simulink model "parallel_two_levelsvpwm"  (R2016a)
settings: Solver=VariableStepAuto  StartTime=0.0  StopTime=0.5  RelTol=1e-3
libraries: powerlib x50, simulink x7, powerlib_meascontrol x2
settings Model: Creator=hakan  LastModifiedBy=hakan
settings DataIOCC: LimitDataPoints=on
settings DebuggingCC: AllowSymbolicDim=off
settings ModelReferenceCC: PropagateSignalLabelsOutOfModel=off
settings GRTTargetCC: GeneratePreprocessorConditionals=Use local settings

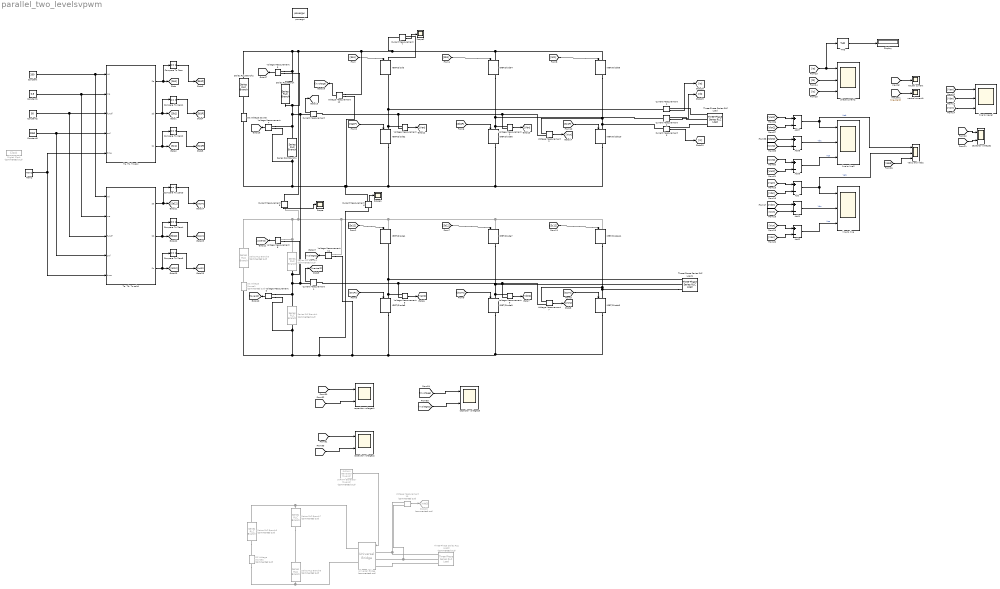
== system parallel_two_levelsvpwm ==
  Add{,1..2,7..9} (6 alike) : Sum  Inputs=+-
  Compare To Zero{,1..5} (6 alike) : simulink/Logic and Bit Operations/Compare To Zero  relop===  OutDataTypeStr=boolean
  Constant : Constant  Value=200
  Constant1 : Constant  Value=0.8
  Constant2 : Constant  Value=50
  Constant3 : Constant  Value=2050  VectorParams1D=off
  Current Measurement{,1..7} (8 alike) : powerlib/Measurements/Current Measurement  PhasorSimulation=off  OutputType=Complex  PSBequivalent=0
  DC Voltage Source : powerlib/Electrical Sources/DC Voltage Source  Amplitude=540  Measurements=None
  DC Voltage Source1 : powerlib/Electrical Sources/DC Voltage Source  Commented=on  Amplitude=540  Measurements=None
  DC Voltage Source2 : powerlib/Electrical Sources/DC Voltage Source  Commented=on  Amplitude=540  Measurements=None
  Digital Clock : DigitalClock  Commented=on  SampleTime=0.0000001
  Display : Display
  Goto28 : Goto  Commented=on  GotoTag=Vab3
  IGBT/Diode{,1..11} (12 alike) : powerlib/Power Electronics/IGBT//Diode  Ron=1e-3  Rs=1e5  Cs=inf  Measurements=on
  Ramp : simulink/Sources/Ramp  slope=1  start=0  X0=0
  SVPWM Generator (2-Level) : powerlib_meascontrol/Pulse & Signal Generators/SVPWM Generator (2-Level)  Commented=on  InputType=Internally generated  SwitchingPattern=Pattern #1  Fc=2050  ParUref="[0.8 0  50]"  Ts=0
  Scope : Scope
  Scope1 : Scope
  Scope2 : Scope
  Series RLC Branch : powerlib/Elements/Series RLC Branch  LConnTagsString=__new0  RConnTagsString=__new0  BranchType=C  Resistance=1  Inductance=1e-3  SetiL0=off  InitialCurrent=0  Capacitance=10e-6  Setx0=off  InitialVoltage=0  Measurements=None
  Series RLC Branch1 : powerlib/Elements/Series RLC Branch  LConnTagsString=__new0  RConnTagsString=__new0  BranchType=C  Resistance=1  Inductance=1e-3  SetiL0=off  InitialCurrent=0  Capacitance=10e-6  Setx0=off  InitialVoltage=0  Measurements=None
  Series RLC Branch2 : powerlib/Elements/Series RLC Branch  LConnTagsString=__new0  RConnTagsString=__new0  BranchType=R  Resistance=1  Inductance=1e-3  SetiL0=off  InitialCurrent=0  Capacitance=1000e-6  Setx0=off  InitialVoltage=0  Measurements=None
  Series RLC Branch3 : powerlib/Elements/Series RLC Branch  Commented=on  LConnTagsString=__new0  RConnTagsString=__new0  BranchType=C  Resistance=1  Inductance=1e-3  SetiL0=off  InitialCurrent=0  Capacitance=10e-6  Setx0=off  InitialVoltage=0  Measurements=None
  Series RLC Branch4 : powerlib/Elements/Series RLC Branch  Commented=on  LConnTagsString=__new0  RConnTagsString=__new0  BranchType=C  Resistance=1  Inductance=1e-3  SetiL0=off  InitialCurrent=0  Capacitance=10e-6  Setx0=off  InitialVoltage=0  Measurements=None
  Series RLC Branch5 : powerlib/Elements/Series RLC Branch  Commented=on  LConnTagsString=__new0  RConnTagsString=__new0  BranchType=R  Resistance=1  Inductance=1e-3  SetiL0=off  InitialCurrent=0  Capacitance=1000e-6  Setx0=off  InitialVoltage=0  Measurements=None
  Series RLC Branch6 : powerlib/Elements/Series RLC Branch  Commented=on  LConnTagsString=__new0  RConnTagsString=__new0  BranchType=R  Resistance=1  Inductance=1e-3  SetiL0=off  InitialCurrent=0  Capacitance=1000e-6  Setx0=off  InitialVoltage=0  Measurements=None
  Series RLC Branch7 : powerlib/Elements/Series RLC Branch  Commented=on  LConnTagsString=__new0  RConnTagsString=__new0  BranchType=C  Resistance=1  Inductance=1e-3  SetiL0=off  InitialCurrent=0  Capacitance=20e-6  Setx0=off  InitialVoltage=0  Measurements=None
  Series RLC Branch8 : powerlib/Elements/Series RLC Branch  Commented=on  LConnTagsString=__new0  RConnTagsString=__new0  BranchType=C  Resistance=1  Inductance=1e-3  SetiL0=off  InitialCurrent=0  Capacitance=20e-6  Setx0=off  InitialVoltage=0  Measurements=None
  THD : powerlib_meascontrol/Measurements/THD  Freq=50  Ts=0
  "Ta, Tb, Tc calc" : MATLAB Function  TreatAsAtomicUnit=on
  "Ta, Tb, Tc calc1" : MATLAB Function  TreatAsAtomicUnit=on
  Three-Phase Series RLC Load : powerlib/Elements/Three-Phase Series RLC Load  LConnTagsString=A|B|C  Configuration=Y (floating)  NominalVoltage=1000  Vabc=[1e3 1e3 1e3]  Vabcp=[1e3 1e3 1e3]  NominalFrequency=50  UnbalancedPower=off  ActivePower=8000/2  InductivePower=3870/2  CapacitivePower=0  Pabc=[10e3 9e3 11e3]  QLabc=[100 90 110]  QCabc=[100 90 110]  Pabcp=[10e3 9e3 11e3]  QLabcp=[100 90 110]  QCabcp=[100 90 110]  Measurements=None  LoadType=constant Z
  Three-Phase Series RLC Load1 : powerlib/Elements/Three-Phase Series RLC Load  LConnTagsString=A|B|C  Configuration=Y (floating)  NominalVoltage=1000  Vabc=[1e3 1e3 1e3]  Vabcp=[1e3 1e3 1e3]  NominalFrequency=50  UnbalancedPower=off  ActivePower=8000/2  InductivePower=3870/2  CapacitivePower=0  Pabc=[10e3 9e3 11e3]  QLabc=[100 90 110]  QCabc=[100 90 110]  Pabcp=[10e3 9e3 11e3]  QLabcp=[100 90 110]  QCabcp=[100 90 110]  Measurements=None  LoadType=constant Z
  Three-Phase Series RLC Load2 : powerlib/Elements/Three-Phase Series RLC Load  Commented=on  LConnTagsString=A|B|C  Configuration=Y (floating)  NominalVoltage=1000  Vabc=[1e3 1e3 1e3]  Vabcp=[1e3 1e3 1e3]  NominalFrequency=50  UnbalancedPower=off  ActivePower=8000/2  InductivePower=3870/2  CapacitivePower=0  Pabc=[10e3 9e3 11e3]  QLabc=[100 90 110]  QCabc=[100 90 110]  Pabcp=[10e3 9e3 11e3]  QLabcp=[100 90 110]  QCabcp=[100 90 110]  Measurements=None  LoadType=constant Z
  Universal Bridge : powerlib/Power Electronics/Universal Bridge  Commented=on  Arms=3  SnubberResistance=1e5  SnubberCapacitance=inf  Device=IGBT / Diodes  Ron=1e-3  Lon=0  ForwardVoltages="[  0  0  ]"  ForwardVoltage=0  GTOparameters=[ 10e-6 , 20e-6 ]  IGBTparameters=[ 1e-6 , 2e-6 ]  Measurements=None  Measurements_2=None  converterType=Rectifier
  Vab1 and Vab2 : Scope  NumInputPorts=3
  Voltage Measurement{,1..9,11..12} (12 alike) : powerlib/Measurements/Voltage Measurement  PhasorSimulation=off  OutputType=Complex  PSBequivalent=0
  Voltage Measurement10 : powerlib/Measurements/Voltage Measurement  Commented=on  PhasorSimulation=off  OutputType=Complex  PSBequivalent=0
  capacitor voltages{,1..3} (4 alike) : Scope  NumInputPorts=2
  line to line : Scope  NumInputPorts=3
  line to line2 : Scope  NumInputPorts=3
  line to neural : Scope  NumInputPorts=3
  neutral current : Scope
  neutral current1 : Scope
  phase currents : Scope  NumInputPorts=3
  powergui : powerlib/powergui  Priority=1  SimulationMode=Discrete  SolverType=Tustin/Backward Euler (TBE)  SampleTime=50e-8  frequency=60  SPID=off  DisableSnubberDevices=off  DisableRonSwitches=off  DisableVfSwitches=off  SwTol=0  DisplayEquations=off  Interpol=off  ExternalGateDelay=off  methode=off  Ts=10  FunctionMessages=off  echomessages=off  HookPort=off  EnableUseOfTLC=off  x0status=blocks  frequencyindice=0  Pbase=100e6  ErrMax=1e-4  Iterations=50  UnitsV=kV  UnitsW=MW  buscounter=0  RestoreLinks=warning  ResistiveCurrentMeasurement=off  Frange=[0:2:500]  Ylog=off  Xlog=on  ShowGrid=off  save=off  variable=ZData  structure=linetoline  ZoomFFT=off  StartTime=0.0  cycles=2  DisplayStyle=1  fundamental=50  FreqAxis=off  MaxFrequency=5000  frequencyindicesteady=1  RmsSteady=1  display=off
  wires:
  "Ta, Tb, Tc calc"/1(Sa) -> Compare To Zero/1, [Sa1]
  "Ta, Tb, Tc calc"/2(Sb) -> Compare To Zero1/1, [Sb1]
  "Ta, Tb, Tc calc"/3(Sc) -> Compare To Zero2/1, [Sc1]
  Compare To Zero/1 -> [Sa1P]
  Compare To Zero1/1 -> [Sb1P]
  Compare To Zero2/1 -> [Sc1P]
  Constant/1 -> "Ta, Tb, Tc calc1"/1(Vd), "Ta, Tb, Tc calc"/1(Vd)
  Constant1/1 -> "Ta, Tb, Tc calc1"/2(ma), "Ta, Tb, Tc calc"/2(ma)
  Constant2/1 -> "Ta, Tb, Tc calc1"/3(fundf), "Ta, Tb, Tc calc"/3(fundf)
  Constant3/1 -> "Ta, Tb, Tc calc1"/4(swf), "Ta, Tb, Tc calc"/4(swf)
  Ramp/1 -> "Ta, Tb, Tc calc"/5(time), "Ta, Tb, Tc calc1"/5(time)
  [Ineutral] -> neutral current/1
  [Ib] -> phase currents/2
  [Ic] -> phase currents/3
  [Van] -> Add/1
  [Vbn] -> Add/2
  Add/1 -> Vab1 and Vab2/2, line to line/1  "Vab"
  [Vbn] -> Add1/1
  [Vcn] -> Add1/2
  Add1/1 -> line to line/2  "Vbc"
  [Vcn] -> Add2/1
  [Van] -> Add2/2
  Add2/1 -> line to line/3  "Vca"
  [Van] -> line to neural/1
  [Vbn] -> line to neural/2
  [Vcn] -> line to neural/3
  [lowerc] -> capacitor voltages/2
  [upperc] -> capacitor voltages/1
  [Sa1] -> IGBT/Diode/1
  [Sa1P] -> IGBT/Diode2/1
  [Sb1] -> IGBT/Diode4/1
  [Sb1P] -> IGBT/Diode6/1
  [Sc1] -> IGBT/Diode8/1
  [Sc1P] -> IGBT/Diode10/1
  Voltage Measurement/1 -> [Van]
  Voltage Measurement1/1 -> [Vbn]
  Voltage Measurement2/1 -> [Vcn]
  Voltage Measurement3/1 -> [upperc]
  Voltage Measurement4/1 -> [lowerc]
  Current Measurement/1 -> [Ineutral]
  Current Measurement1/1 -> [Ia]
  Current Measurement2/1 -> [Ib]
  Current Measurement3/1 -> [Ic]
  "Ta, Tb, Tc calc1"/1(Sa) -> [Sa12], Compare To Zero3/1
  "Ta, Tb, Tc calc1"/2(Sb) -> [Sb12], Compare To Zero4/1
  "Ta, Tb, Tc calc1"/3(Sc) -> [Sc12], Compare To Zero5/1
  Compare To Zero3/1 -> [Sa1P2]
  Compare To Zero4/1 -> [Sb1P2]
  Compare To Zero5/1 -> [Sc1P2]
  [Sa12] -> IGBT/Diode1/1
  [Sa1P2] -> IGBT/Diode5/1
  [Sb12] -> IGBT/Diode7/1
  [Sb1P2] -> IGBT/Diode9/1
  [Sc12] -> IGBT/Diode11/1
  [Sc1P2] -> IGBT/Diode3/1
  Voltage Measurement5/1 -> [Van2]
  Voltage Measurement6/1 -> [Vbn2]
  Voltage Measurement7/1 -> [Vcn2]
  Voltage Measurement8/1 -> [upperc2]
  Voltage Measurement9/1 -> [lowerc2]
  Current Measurement4/1 -> [Ineutral2]
  Voltage Measurement11/1 -> [involtage2]
  [Van2] -> Add7/1
  [Vbn2] -> Add7/2
  Add7/1 -> Vab1 and Vab2/1, line to line2/1  "Vab"
  [Vbn2] -> Add8/1
  [Vcn2] -> Add8/2
  Add8/1 -> line to line2/2  "Vbc"
  [Vcn2] -> Add9/1
  [Van2] -> Add9/2
  Add9/1 -> line to line2/3  "Vca"
  [upperc] -> capacitor voltages1/1
  [lowerc] -> capacitor voltages2/1
  [upperc2] -> capacitor voltages1/2
  [lowerc2] -> capacitor voltages2/2
  [involtage] -> capacitor voltages3/1
  [involtage2] -> capacitor voltages3/2
  [Ineutral2] -> neutral current1/1
  SVPWM Generator (2-Level)/1 -> Universal Bridge/1
  Voltage Measurement10/1 -> Goto28/1
  [Vab3] -> Vab1 and Vab2/3
  Voltage Measurement12/1 -> [involtage]
  [Ia] -> THD/1, phase currents/1
  THD/1 -> Display/1
  Current Measurement5/1 -> Scope/1
  Current Measurement6/1 -> Scope1/1
  Current Measurement7/1 -> Scope2/1
  connections:
  Series RLC Branch5/LConn1 -- Voltage Measurement11/LConn1 -- IGBT/Diode1/LConn1 -- IGBT/Diode11/LConn1 -- IGBT/Diode7/LConn1 -- Current Measurement5/RConn1 -- Voltage Measurement8/LConn1 -- Series RLC Branch3/LConn1
  Current Measurement1/LConn1 -- IGBT/Diode/RConn1 -- IGBT/Diode2/LConn1 -- Voltage Measurement/LConn1
  Current Measurement/LConn1 -- Voltage Measurement/LConn2 -- Voltage Measurement2/LConn2 -- Voltage Measurement1/LConn2
  Current Measurement2/LConn1 -- IGBT/Diode4/RConn1 -- IGBT/Diode6/LConn1 -- Voltage Measurement1/LConn1
  Voltage Measurement2/LConn1 -- IGBT/Diode10/LConn1 -- Current Measurement3/LConn1 -- IGBT/Diode8/RConn1
  Three-Phase Series RLC Load/LConn3 -- Current Measurement3/RConn1
  Three-Phase Series RLC Load/LConn1 -- Current Measurement1/RConn1
  Three-Phase Series RLC Load/LConn2 -- Current Measurement2/RConn1
  DC Voltage Source/RConn1 -- Series RLC Branch2/RConn1
  IGBT/Diode5/LConn1 -- IGBT/Diode1/RConn1 -- Three-Phase Series RLC Load1/LConn1 -- Voltage Measurement5/LConn1
  Voltage Measurement7/LConn2 -- Voltage Measurement6/LConn2 -- Current Measurement4/LConn1 -- Voltage Measurement5/LConn2
  IGBT/Diode9/LConn1 -- IGBT/Diode7/RConn1 -- Three-Phase Series RLC Load1/LConn2 -- Voltage Measurement6/LConn1
  Three-Phase Series RLC Load1/LConn3 -- IGBT/Diode3/LConn1 -- Voltage Measurement7/LConn1 -- IGBT/Diode11/RConn1
  DC Voltage Source1/RConn1 -- Series RLC Branch5/RConn1
  Current Measurement6/RConn1 -- IGBT/Diode2/RConn1 -- IGBT/Diode10/RConn1 -- IGBT/Diode6/RConn1 -- Voltage Measurement12/LConn2 -- Series RLC Branch1/RConn1 -- Voltage Measurement4/LConn2 -- DC Voltage Source/LConn1
  Three-Phase Series RLC Load2/LConn1 -- Universal Bridge/LConn1 -- Voltage Measurement10/LConn1
  Three-Phase Series RLC Load2/LConn2 -- Universal Bridge/LConn2 -- Voltage Measurement10/LConn2
  Three-Phase Series RLC Load2/LConn3 -- Universal Bridge/LConn3
  Series RLC Branch6/RConn1 -- DC Voltage Source2/RConn1
  Series RLC Branch7/RConn1 -- Series RLC Branch8/LConn1
  Series RLC Branch6/LConn1 -- Universal Bridge/RConn1 -- Series RLC Branch7/LConn1
  DC Voltage Source2/LConn1 -- Universal Bridge/RConn2 -- Series RLC Branch8/RConn1
  Voltage Measurement8/LConn2 -- Series RLC Branch3/RConn1 -- Current Measurement4/RConn1 -- Series RLC Branch/RConn1 -- Voltage Measurement3/LConn2 -- Voltage Measurement4/LConn1 -- Series RLC Branch1/LConn1 -- Current Measurement/RConn1 -- Voltage Measurement9/LConn1 -- Series RLC Branch4/LConn1
  Voltage Measurement11/LConn2 -- Voltage Measurement9/LConn2 -- Series RLC Branch4/RConn1 -- DC Voltage Source1/LConn1 -- Current Measurement6/LConn1 -- IGBT/Diode9/RConn1 -- IGBT/Diode3/RConn1 -- IGBT/Diode5/RConn1
  IGBT/Diode/LConn1 -- Current Measurement7/RConn1
  Voltage Measurement12/LConn1 -- Current Measurement7/LConn1 -- IGBT/Diode4/LConn1 -- IGBT/Diode8/LConn1 -- Current Measurement5/LConn1 -- Series RLC Branch2/LConn1 -- Voltage Measurement3/LConn1 -- Series RLC Branch/LConn1

== matlab function parallel_two_levelsvpwm/Ta, Tb, Tc calc ==
  data: Sa output; Sb output; Vd input; ma input; fundf input; swf input; time input; Sc output
function [Sa, Sb, Sc] = fcn(Vd,ma,fundf, swf, time)
% this program works for magnitude of Vref is greater then Vd/3 meaning ma
% must be greater than 1/sqrt(3). for smaller ma's computation is a bit
% more tricky therefore it is omitted for simplicity for now. 
Vref = ma*Vd/sqrt(3); %magnitude of Vref
theta = 2*pi*fundf*time; %angle of Vref
angle = mod(theta, 2*pi);
Ts = 1/swf;
Ta = 0;
Tb = 0;
Tc = 0;
T0 = 0;
n=0;
output = 0;
%Sector1 = 0; Sector2 = 0; Sector3 = 0; Sector4= 0; Sector5 = 0; Sector6 = 0;
Sa=0; Sb=0; Sc=0;
timee = mod(time,Ts);



%% Sector 1
if (angle<=pi/3)&&(angle>0)  % sector 1
    n = 1;
    thetaprime = angle - (n-1)*pi/3;
    
    Ta = Ts*ma*sin(pi/3-thetaprime);
    Tb = Ts*ma*sin(thetaprime);
    T0 = Ts-Ta-Tb;
    
    times = [T0/4 Tb/2 Ta/2 T0/2 Ta/2 Tb/2 T0/4];
    times = cumsum(times);
    va= [0 1 1 1 1 1 0];
    vb= [0 0 1 1 1 0 0];
    vc= [0 0 0 1 0 0 0];
    
    for j = 1:7            
            if(timee<times(j))
                break
            end
    end
        Sa=va(j); 
        Sb=vb(j); 
        Sc=vc(j); 
end
%% Sector 2
if (angle<=2*pi/3)&&(angle>pi/3)  % sector 2
    n = 2;
    thetaprime = angle - (n-1)*pi/3;
    
    Ta = Ts*ma*sin(pi/3-thetaprime);
    Tb = Ts*ma*sin(thetaprime);
    T0 = Ts-Ta-Tb;   
    
    times = [T0/4 Tb/2 Ta/2 T0/2 Ta/2 Tb/2 T0/4];
    times = cumsum(times);
    va= [0 0 1 1 1 0 0];
    vb= [0 1 1 1 1 1 0];
    vc= [0 0 0 1 0 0 0];
    
    for j = 1:7            
            if(timee<times(j))
                break
            end
    end
        Sa=va(j); 
        Sb=vb(j); 
        Sc=vc(j); 
end


%% Sector 3
if (angle<=pi)&&(angle>2*pi/3)  % sector 3
    n = 3;
    thetaprime = angle - (n-1)*pi/3;
    
    Ta = Ts*ma*sin(pi/3-thetaprime);
    Tb = Ts*ma*sin(thetaprime);
    T0 = Ts-Ta-Tb;  
    
    times = [T0/4 Tb/2 Ta/2 T0/2 Ta/2 Tb/2 T0/4];
    times = cumsum(times);
    va= [0 0 0 1 0 0 0];
    vb= [0 1 1 1 1 1 0];
    vc= [0 0 1 1 1 0 0];
    
    for j = 1:7            
            if(timee<times(j))
                break
            end
    end
        Sa=va(j); 
        Sb=vb(j); 
        Sc=vc(j);     
end


%% Sector 4
if (angle<=4*pi/3)&&(angle>pi)  % sector 4
    n = 4;
    thetaprime = angle - (n-1)*pi/3;
    
    Ta = Ts*ma*sin(pi/3-thetaprime);
    Tb = Ts*ma*sin(thetaprime);
    T0 = Ts-Ta-Tb;
    
    times = [T0/4 Tb/2 Ta/2 T0/2 Ta/2 Tb/2 T0/4];
    times = cumsum(times);
    va = [0 0 0 1 0 0 0];
    vb = [0 0 1 1 1 0 0];
    vc = [0 1 1 1 1 1 0];
    
    for j = 1:7            
            if(timee<times(j))
                break
            end
    end
        Sa=va(j); 
        Sb=vb(j); 
        Sc=vc(j); 
    
end


%% Sector 5 
if (angle<=5*pi/3)&&(angle>4*pi/3)  % sector 5
    n = 5;
    thetaprime = angle - (n-1)*pi/3;
    
    Ta = Ts*ma*sin(pi/3-thetaprime);
    Tb = Ts*ma*sin(thetaprime);
    T0 = Ts-Ta-Tb;
    
    times = [T0/4 Tb/2 Ta/2 T0/2 Ta/2 Tb/2 T0/4];
    times = cumsum(times);
    va= [0 0 1 1 1 0 0];
    vb= [0 0 0 1 0 0 0];
    vc= [0 1 1 1 1 1 0];
    
    for j = 1:7            
            if(timee<times(j))
                break
            end
    end
        Sa=va(j); 
        Sb=vb(j); 
        Sc=vc(j); 
    
end


%% Sector 6 
if (angle<=2*pi)&&(angle>5*pi/3)  % sector 6
    n = 6;
    thetaprime = angle - (n-1)*pi/3;
    
    Ta = Ts*ma*sin(pi/3-thetaprime);
    Tb = Ts*ma*sin(thetaprime);
    T0 = Ts-Ta-Tb;
    
    times = [T0/4 Tb/2 Ta/2 T0/2 Ta/2 Tb/2 T0/4];
    times = cumsum(times);
    va= [0 1 1 1 1 1 0];
    vb= [0 0 0 1 0 0 0];
    vc= [0 0 1 1 1 0 0];
    
    
    for j = 1:7            
            if(timee<times(j))
                break
            end
    end
        Sa=va(j); 
        Sb=vb(j); 
        Sc=vc(j); 
end

== matlab function parallel_two_levelsvpwm/Ta, Tb, Tc calc1 ==
  data: Sa output; Sb output; Vd input; ma input; fundf input; swf input; time input; Sc output
function [Sa, Sb, Sc] = fcn(Vd,ma,fundf, swf, time)
% this program works for magnitude of Vref is greater then Vd/3 meaning ma
% must be greater than 1/sqrt(3). for smaller ma's computation is a bit
% more tricky therefore it is omitted for simplicity for now. 
Vref = ma*Vd/sqrt(3); %magnitude of Vref
theta = 2*pi*fundf*time; %angle of Vref
angle = mod(theta, 2*pi);
Ts = 1/swf;
Ta = 0;
Tb = 0;
Tc = 0;
T0 = 0;
n=0;
output = 0;
%Sector1 = 0; Sector2 = 0; Sector3 = 0; Sector4= 0; Sector5 = 0; Sector6 = 0;
Sa=0; Sb=0; Sc=0;
timee = mod(time+Ts/4,Ts);



%% Sector 1
if (mod(theta, 2*pi)<=pi/3)&&(mod(theta, 2*pi)>0)  % sector 1
    n = 1;
    thetaprime = angle - (n-1)*pi/3;
    
    Ta = Ts*ma*sin(pi/3-thetaprime);
    Tb = Ts*ma*sin(thetaprime);
    T0 = Ts-Ta-Tb;
    
    times = [T0/4 Tb/2 Ta/2 T0/2 Ta/2 Tb/2 T0/4];
    times = cumsum(times);
    va= [0 1 1 1 1 1 0];
    vb= [0 0 1 1 1 0 0];
    vc= [0 0 0 1 0 0 0];
    
    for j = 1:7            
            if(timee<times(j))
                break
            end
    end
        Sa=va(j); 
        Sb=vb(j); 
        Sc=vc(j); 
end
%% Sector 2
if (mod(theta, 2*pi)<=2*pi/3)&&(mod(theta, 2*pi)>pi/3)  % sector 2
    n = 2;
    thetaprime = angle - (n-1)*pi/3;
    
    Ta = Ts*ma*sin(pi/3-thetaprime);
    Tb = Ts*ma*sin(thetaprime);
    T0 = Ts-Ta-Tb;   
    
    times = [T0/4 Tb/2 Ta/2 T0/2 Ta/2 Tb/2 T0/4];
    times = cumsum(times);
    va= [0 0 1 1 1 0 0];
    vb= [0 1 1 1 1 1 0];
    vc= [0 0 0 1 0 0 0];
    
    for j = 1:7            
            if(timee<times(j))
                break
            end
    end
        Sa=va(j); 
        Sb=vb(j); 
        Sc=vc(j); 
end


%% Sector 3
if (mod(theta, 2*pi)<=pi)&&(mod(theta, 2*pi)>2*pi/3)  % sector 3
    n = 3;
    thetaprime = angle - (n-1)*pi/3;
    
    Ta = Ts*ma*sin(pi/3-thetaprime);
    Tb = Ts*ma*sin(thetaprime);
    T0 = Ts-Ta-Tb;  
    
    times = [T0/4 Tb/2 Ta/2 T0/2 Ta/2 Tb/2 T0/4];
    times = cumsum(times);
    va= [0 0 0 1 0 0 0];
    vb= [0 1 1 1 1 1 0];
    vc= [0 0 1 1 1 0 0];
    
    for j = 1:7            
            if(timee<times(j))
                break
            end
    end
        Sa=va(j); 
        Sb=vb(j); 
        Sc=vc(j);     
end


%% Sector 4
if (mod(theta, 2*pi)<=4*pi/3)&&(mod(theta, 2*pi)>pi)  % sector 4
    n = 4;
    thetaprime = angle - (n-1)*pi/3;
    
    Ta = Ts*ma*sin(pi/3-thetaprime);
    Tb = Ts*ma*sin(thetaprime);
    T0 = Ts-Ta-Tb;
    
    times = [T0/4 Tb/2 Ta/2 T0/2 Ta/2 Tb/2 T0/4];
    times = cumsum(times);
    va = [0 0 0 1 0 0 0];
    vb = [0 0 1 1 1 0 0];
    vc = [0 1 1 1 1 1 0];
    
    for j = 1:7            
            if(timee<times(j))
                break
            end
    end
        Sa=va(j); 
        Sb=vb(j); 
        Sc=vc(j); 
    
end


%% Sector 5 
if (mod(theta, 2*pi)<=5*pi/3)&&(mod(theta, 2*pi)>4*pi/3)  % sector 5
    n = 5;
    thetaprime = angle - (n-1)*pi/3;
    
    Ta = Ts*ma*sin(pi/3-thetaprime);
    Tb = Ts*ma*sin(thetaprime);
    T0 = Ts-Ta-Tb;
    
    times = [T0/4 Tb/2 Ta/2 T0/2 Ta/2 Tb/2 T0/4];
    times = cumsum(times);
    va= [0 0 1 1 1 0 0];
    vb= [0 0 0 1 0 0 0];
    vc= [0 1 1 1 1 1 0];
    
    for j = 1:7            
            if(timee<times(j))
                break
            end
    end
        Sa=va(j); 
        Sb=vb(j); 
        Sc=vc(j); 
    
end


%% Sector 6 
if (mod(theta, 2*pi)<=2*pi)&&(mod(theta, 2*pi)>5*pi/3)  % sector 6
    n = 6;
    thetaprime = angle - (n-1)*pi/3;
    
    Ta = Ts*ma*sin(pi/3-thetaprime);
    Tb = Ts*ma*sin(thetaprime);
    T0 = Ts-Ta-Tb;
    
    times = [T0/4 Tb/2 Ta/2 T0/2 Ta/2 Tb/2 T0/4];
    times = cumsum(times);
    va= [0 1 1 1 1 1 0];
    vb= [0 0 0 1 0 0 0];
    vc= [0 0 1 1 1 0 0];
    
    
    for j = 1:7            
            if(timee<times(j))
                break
            end
    end
        Sa=va(j); 
        Sb=vb(j); 
        Sc=vc(j); 
end
